simulink model "synapse_with_facilitation"  (R2022a)
settings: Solver=VariableStepAuto  StartTime=0.0  StopTime=10000  RelTol=1e-3
libraries: simulink x4, neuromorphic_blocks x4
settings Model: Creator=chris  LastModifiedBy=chris

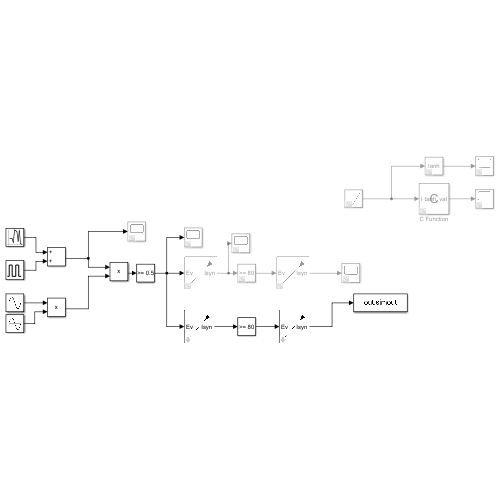
[thumbnail: Simulink's stored preview of the top-level diagram]
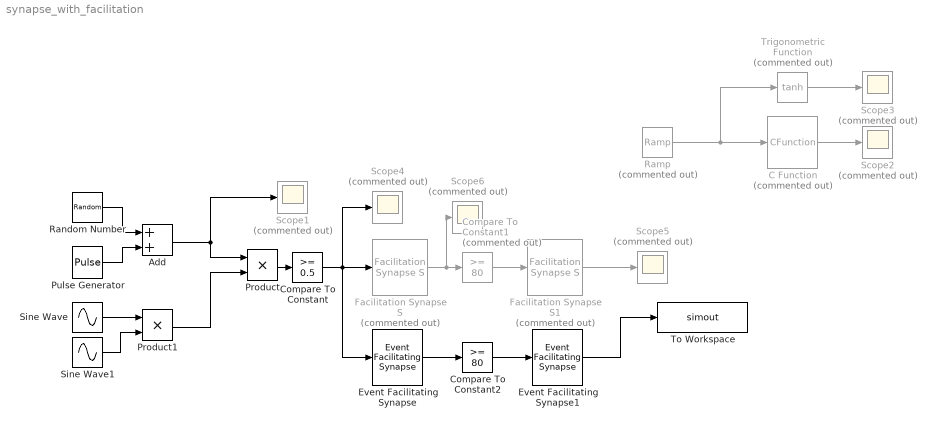
== system synapse_with_facilitation ==
  Add : Sum
  C Function : CFunction  Commented=on  OutputCode=|
      | if (I < -4.971786858528029) {
      |     tanh_val = -1;
      | } else {
      | if (I > 4.971786858528029) {
      |     tanh_val = 1;
      | } else {
      |     double x2 = I * I;
      |     double a = I * (135135.0 + x2 * (17325.0 + x2 * (378.0 + x2)));
      |     double b = 135135.0 + x2 * (62370.0 + x2 * (3150.0 + x2 * 28.0));
      |     tanh_val = a / b;
      | }
      | }
  Compare To Constant : simulink/Logic and Bit Operations/Compare To Constant  relop=>=  const=0.5  OutDataTypeStr=boolean
  Compare To Constant1 : simulink/Logic and Bit Operations/Compare To Constant  Commented=on  relop=>=  const=80  OutDataTypeStr=boolean
  Compare To Constant2 : simulink/Logic and Bit Operations/Compare To Constant  relop=>=  const=80  OutDataTypeStr=boolean
  Event Facilitating Synapse : neuromorphic_blocks/Events Transmission Blocks/Event Facilitating Synapse  gsyn_source=Internal  gsyn=100  dsyn=2.5  msyn=5  timescale=0.004  rel_timescale=10
  Event Facilitating Synapse1 : neuromorphic_blocks/Events Transmission Blocks/Event Facilitating Synapse  gsyn_source=Internal  gsyn=100  dsyn=2.5  msyn=5  timescale=0.004  rel_timescale=10
  Facilitation Synapse S : neuromorphic_blocks/Facilitation Synapse S  Commented=on  gsyn_source=Internal  gsyn=100  dsyn=2.5  msyn=5  timescale=0.004  rel_timescale=10  voltage_input=off  gsyn_in=0  dsyn_in=0  msyn_in=1
      settings: SourceProductName=Neuromorphic Toolbox
  Facilitation Synapse S1 : neuromorphic_blocks/Facilitation Synapse S  Commented=on  gsyn_source=Internal  gsyn=100  dsyn=2.5  msyn=5  timescale=0.004  rel_timescale=10  voltage_input=off  gsyn_in=0  dsyn_in=0  msyn_in=1
      settings: SourceProductName=Neuromorphic Toolbox
  Product : Product
  Product1 : Product
  Pulse Generator : DiscretePulseGenerator  PulseType=Time based  Period=0.05  PulseWidth=60  PhaseDelay=0.01
  Ramp : simulink/Sources/Ramp  Commented=on  slope=1  start=0  InitialOutput=-5
  Random Number : RandomNumber  Variance=0.5  SampleTime=0.01
  Scope{1..6} (6 alike) : Scope  Commented=on
  Sine Wave : Sin  Amplitude=0.5  Bias=0.5  Frequency=3  SampleTime=0
  Sine Wave1 : Sin  Amplitude=0.5  Bias=0.5  Frequency=3.5  SampleTime=0
  To Workspace : ToWorkspace  VariableName=simout  SaveFormat=Timeseries  SampleTime=-1
  Trigonometric Function : Trigonometry  Commented=on  Operator=tanh
  wires:
  C Function/1 -> Scope2/1
  Ramp/1 -> Trigonometric Function/1, C Function/1
  Trigonometric Function/1 -> Scope3/1
  Compare To Constant/1 -> Event Facilitating Synapse/1, Scope4/1, Facilitation Synapse S/1
  Product/1 -> Compare To Constant/1
  Sine Wave/1 -> Product1/1
  Sine Wave1/1 -> Product1/2
  Product1/1 -> Product/2
  Add/1 -> Product/1, Scope1/1
  Pulse Generator/1 -> Add/2
  Random Number/1 -> Add/1
  Facilitation Synapse S/1 -> Scope6/1, Compare To Constant1/1
  Compare To Constant1/1 -> Facilitation Synapse S1/1
  Event Facilitating Synapse/1 -> Compare To Constant2/1
  Compare To Constant2/1 -> Event Facilitating Synapse1/1
  Facilitation Synapse S1/1 -> Scope5/1
  Event Facilitating Synapse1/1 -> To Workspace/1
